simulink model "hbridge"  (R2017a)
settings: Solver=VariableStepAuto  StartTime=0.0  StopTime=1/250  MaxStep=1e-4  RelTol=1e-3
libraries: powerlib x12, powerlib_meascontrol x2
settings Model: Creator=gabriel  LastModifiedBy=gabriel

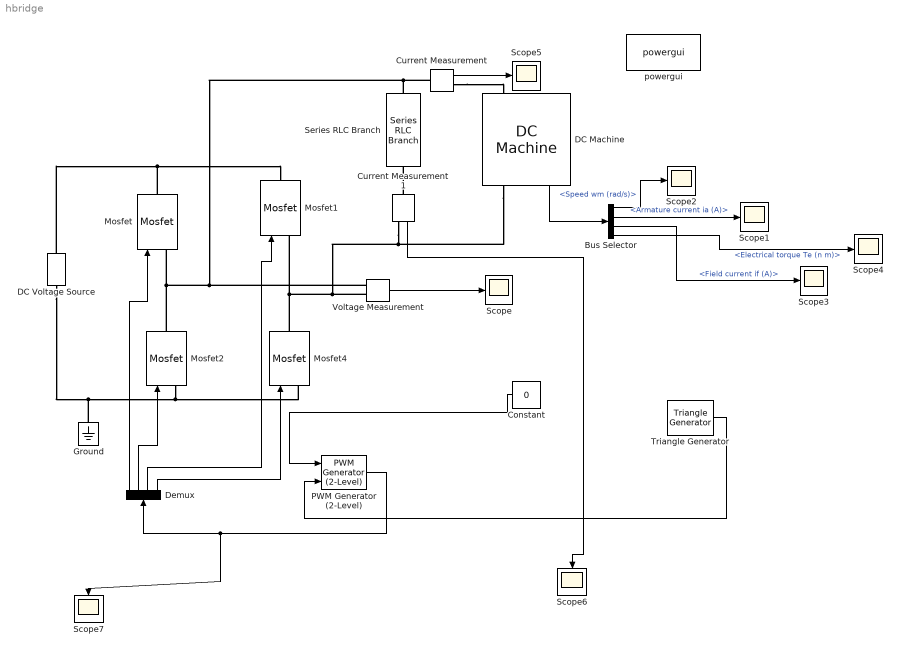
== system hbridge ==
  Bus Selector : BusSelector  OutputSignals=Speed wm (rad/s),Armature current ia (A),Field current if (A),Electrical torque Te (n m)
  Constant : Constant  Value=0
  Current Measurement : powerlib/Measurements/Current Measurement  PhasorSimulation=off  OutputType=Complex  PSBequivalent=0
  Current Measurement1 : powerlib/Measurements/Current Measurement  PhasorSimulation=off  OutputType=Complex  PSBequivalent=0
  DC Machine : powerlib/Machines/DC Machine  PresetModel=No  MechanicalLoad=Torque TL  FieldType=Permanent magnet  ShowDetailedParameters=on  MeasurementBus=off  RLa=[ 1.07 0.05]  RLf="[ 240  120]"  Laf=1.8  MachineConstant=Torque constant (N.m/A)  Ke=1.8  Kt=3.41  J=1.5*10^-8  Bm=4*10^-7  Tf=0  w0=0  Ifinit=0  TsPowergui=0  TsBlock=-1
  DC Voltage Source : powerlib/Electrical Sources/DC Voltage Source  Amplitude=18  Measurements=Voltage
  Demux : Demux
  Ground : powerlib/Elements/Ground  LConnTagsString=a
  Mosfet{,1..2,4} (4 alike) : powerlib/Power Electronics/Mosfet  Ron=0.1  Lon=0  Rd=0.01  Vfd=0  IC=0  Rs=1e5  Cs=inf  Measurements=off
  PWM Generator (2-Level) : powerlib_meascontrol/Pulse & Signal Generators/PWM Generator (2-Level)  ModulatorType=Single-phase full-bridge - Bipolar modulation (4 pulses)  ModulatorMode=Synchronized  Fc=1000  Pc=90  nF=1  MinMax=[ -1 1 ]  SamplingTechnique=Natural  ModulatingSignals=off  m=0.8  Freq=60  Phase=0  Ts=0  ShowCarrierOutport=off
      settings: SourceProductName=Simscape Power Systems
  Scope{,1..7} (8 alike) : Scope
  Series RLC Branch : powerlib/Elements/Series RLC Branch  LConnTagsString=__new0  RConnTagsString=__new0  BranchType=C  Resistance=1  Inductance=1e-3  SetiL0=off  InitialCurrent=0  Capacitance=1e-2  Setx0=off  InitialVoltage=0  Measurements=None
  Triangle Generator : powerlib_meascontrol/Pulse & Signal Generators/Triangle Generator  Freq=1000  Phase=90  Ts=0
  Voltage Measurement : powerlib/Measurements/Voltage Measurement  PhasorSimulation=off  OutputType=Complex  PSBequivalent=0
  powergui : powerlib/powergui  Priority=1  SimulationMode=Continuous  SampleTime=50e-6  frequency=60  Iterations=50  frequencyindice=0  Pbase=100e6  ErrMax=1e-4  UnitsV=kV  UnitsW=MW  buscounter=0  FunctionMessages=off  echomessages=off  EnableUseOfTLC=off  CurrentSourceSwitches=off  DisableSnubberDevices=off  DisableRonSwitches=off  DisableVfSwitches=off  DisplayEquations=off  SolverType=Tustin/Backward Euler (TBE)  Interpol=off  ExternalGateDelay=off  methode=off  Ts=100  x0status=blocks  SPID=on  SwTol=0  HookPort=off  RestoreLinks=warning  ResistiveCurrentMeasurement=off  Frange=[0:2:500]  Ylog=off  Xlog=on  ShowGrid=off  save=off  variable=ZData  structure=0  ZoomFFT=off  StartTime=0.0  cycles=1  DisplayStyle=1  fundamental=60  FreqAxis=off  MaxFrequency=1000  frequencyindicesteady=1  RmsSteady=1  display=off
  wires:
  PWM Generator (2-Level)/1 -> Scope7/1, Demux/1
  Voltage Measurement/1 -> Scope/1
  Triangle Generator/1 -> PWM Generator (2-Level)/2
  Constant/1 -> PWM Generator (2-Level)/1
  DC Machine/1 -> Bus Selector/1
  Bus Selector/1 -> Scope2/1  "<Speed wm (rad/s)>"
  Bus Selector/2 -> Scope1/1  "<Armature current ia (A)>"
  Bus Selector/3 -> Scope3/1  "<Field current if (A)>"
  Bus Selector/4 -> Scope4/1  "<Electrical torque Te (n m)>"
  Current Measurement/1 -> Scope5/1
  Current Measurement1/1 -> Scope6/1
  Demux/1 -> Mosfet/1
  Demux/2 -> Mosfet2/1
  Demux/3 -> Mosfet1/1
  Demux/4 -> Mosfet4/1
  connections:
  Mosfet2/RConn1 -- Current Measurement/LConn1 -- Series RLC Branch/LConn1 -- Voltage Measurement/LConn1 -- Mosfet/LConn1
  Mosfet4/RConn1 -- Current Measurement1/RConn1 -- DC Machine/RConn1 -- Voltage Measurement/LConn2 -- Mosfet1/LConn1
  Mosfet/RConn1 -- DC Voltage Source/RConn1 -- Mosfet1/RConn1
  Mosfet2/LConn1 -- DC Voltage Source/LConn1 -- Ground/LConn1 -- Mosfet4/LConn1
  Current Measurement/RConn1 -- DC Machine/LConn1
  Current Measurement1/LConn1 -- Series RLC Branch/RConn1
